simulink model "NLGuidance"  (R2016a)
settings: Solver=ode3  StartTime=0.0  StopTime=10.0  FixedStep=.02  RelTol=1e-3
model workspace (MAT data in the model file):
  F = [0.0104799567177; 0.0105274136759; 0.00258730184958; 0.00112291450915; 0.0065543125439; 0]
  N = 51
  S1 = [2.42464759278 -2.49697623385 -0.253883104432 -3.312058597 3.28063521535 2.42464759278 -2.49697623385 -0.253883104432 -3.312058597 3.28063521535 2.42464759278 -2.49697623385 ... (7515 elements, 5x1503)]
  S2 = [-47.5753524072 -52.4969762338 -50.2538831044 -53.312058597 -46.7193647847 -53.1933464928 -58.0206597562 -53.298625948 -53.0732596071 -45.5277132009 -58.8093605499 -63.5421671216 ... (7515 elements, 5x1503)]
  S3 = [-5.62481372887 -5.52769980874 -3.05143765206 0.237149289911 1.1849461568 -5.61799408553 -5.52368352234 -3.04474284358 0.238798989919 1.19165158379 -5.61601405716 -5.52150736543 ... (7515 elements, 5x1503)]
  S4 = [0 0 0 0 0 0 0 0 0 0 0 0 ... (7515 elements, 5x1503)]
  Vt = [0 0 0 0 0 0 0 0 0 0 0 0 ... (1503 elements, 501x3)]
  Vv = [1.1849461568 1.19165158379 1.19363427504 1.1947051518 1.20742767257 1.21177592763 1.21717805586 1.22205358332 1.22753574851 1.22892415591 1.22911717004 1.25058652202 ... (1503 elements, 501x3)]
  Vvmag = [6.45855507903 6.44973720458 6.44685088198 6.4408859639 6.4366826743 6.42659096353 6.42411891458 6.41278379056 6.40944425236 6.4051659263 6.38964384833 6.38667032718 ... (501 elements, 501x1)]
  X = [2.42464759278  -3.58806283515  -3.13212037163  -4.62859462973  -4.56044848222  -1.58805327826  -4.31562089748  -1.59798361729  3.6518933724  -1.65480947533  1.86919995453  -3.44104646715; -2.49697623385  -3.26410626081  1.1374607513  -4.53307798606  3.16641265871  2.30316995677  -4.22846546614  1.19685177791  4.5962066329  1.482802268  -2.27100282896  -2.50278022892; -0.253883104432  1.58732884776  -3.37955300207  -2.05245406097  -2.56581901551  -2.72520301408  -1.22048178872  -1.58600952642  3.65490458678  1.85411206404  -0.00605968294054  -1.90223108815; -3.312058597  1.68742830515  3.12131217871  1.23610531908  3.08830453111  -2.73426128729  -0.852168562096  1.63529528737  1.04129979322  3.9147593874  -2.83132054006  -1.00180163899; 3.28063521535  1.89810778603  4.32221989343  2.18269243779  -3.3024120093  -2.00531011718  -0.0516837044744  2.44755242786  1.9309412878  5  4.9501252848  -0.842692668272; -3.6978315289  -3.58806283515  1.68549199744  -4.5188954159  -4.66205440883  -1.6875649026  -4.35220746466  1.34311705486  0.811657546537  -1.85555021076  -3.19980711127  -4.38418451801]
  Xap1 = [3.53742766553 3.54841812521 3.55649436401 3.56301032299 3.56900127601 3.57285766144 3.57579889741 3.57816116305 3.57954580685 3.57954139291 3.5792899619 3.58161806007 ... (1503 elements, 501x3)]
  Xap2 = [3.00894026262 2.99947384008 2.99278206158 2.98751350515 2.98264302934 2.97978827516 2.97774180284 2.97617755456 2.97550435147 2.97614326838 2.97696071264 2.97513994677 ... (1503 elements, 501x3)]
  Xr = [10 11.2284720857 12.4539847001 13.6735561742 14.8879723634 16.0937793652 17.2959786101 18.4820399899 19.6645679603 20.8393619799 21.9947001613 23.1446286766 ... (1503 elements, 501x3)]
  Xrmag = [15.65732221 23.8105907731 30.9856356907 38.4540834067 46.0738528973 53.7662892745 61.5065103501 69.2725920166 77.0607192366 84.8582850512 92.6527324163 100.450411961 ... (501 elements, 501x1)]
  Xtarg = [3.28063521535 3.28063521535 3.28063521535 3.28063521535 3.28063521535 3.28063521535 3.28063521535 3.28063521535 3.28063521535 3.28063521535 3.28063521535 3.28063521535 ... (1503 elements, 501x3)]
  Xv = [-46.7193647847 -45.5277132009 -44.3340789258 -43.139373774 -41.9319461015 -40.7201701738 -39.502992118 -38.2809385346 -37.0534027861 -35.8244786302 -34.5953614602 -33.3447749382 ... (1503 elements, 501x3)]
  ans = [0  0  0; 2  2  2; 4  4  4]
  cmd = timeseries
  cmd.DataInfo = tsdata.datametadata
  cmd.DataInfo.Interpolation = tsdata.interpolation
  cmd.DataInfo.Interpolation.Fhandle : function handle (value not decoded)
  cmd.DataInfo.Interpolation.Name = 'zoh'
  cmd.TimeInfo = tsdata.timemetadata
  cmd.TimeInfo.DuplicateTimes = 0
  cmd.TimeInfo.Initialized = 1
  cmd.QualityInfo = tsdata.qualmetadata
  cmd1 = []
  cmd2 = []
  count = 136
  curPath = '/Users/khouloud.gaaloul/Documents/Projects/QRA-Search/Problems/SimulinkTesting'
  curve : matlab.graphics.animation.AnimatedLine (value not decoded)
  curveo = matlab.graphics.animation.AnimatedLine
  curveo.LineWidthMode = 'manual'
  curveo.LineWidth_I = 2
  curveo.CurrentLine_I = 0
  curveo.SegmentContainer_I = matlab.graphics.primitive.world.Group
  curveo.SegmentContainer_I.SerializableChildren = matlab.graphics.internal.AnimatedSegment
  curveo.SegmentContainer_I.SerializableChildren.Edge = matlab.graphics.primitive.world.LineStrip
  curveo.SegmentContainer_I.SerializableChildren.Edge.StripData_I = [1 502]
  curveo.SegmentContainer_I.SerializableChildren.Edge.LineWidth_I = 2
  curveo.SegmentContainer_I.SerializableChildren.Edge.VertexData_I = [3.00894021988 2.64835071564 4.92497825623 2.9994738102 2.63493180275 4.93706846237 2.99278211594 2.62207984924 4.94912099838 2.98751354218 2.61010932922 4.96028995514 ... (1503 elements, 3x501)]
  curveo.SegmentContainer_I.SerializableChildren.Edge.ColorData_I = [0; 0; 0; 255]
  curveo.SegmentContainer_I.SerializableChildren.Edge.ColorBinding_I = 'object'
  curveo.SegmentContainer_I.SerializableChildren.Edge.Description_I = 'AnimatedSegment Edge'
  curveo.SegmentContainer_I.SerializableChildren.Edge.HandleVisibility_I = 'off'
  curveo.SegmentContainer_I.SerializableChildren.Edge.Internal = 1
  curveo.SegmentContainer_I.SerializableChildren.Edge.SerializableApplicationData = struct()
  curveo.SegmentContainer_I.SerializableChildren.Edge.Copyable = 1
  curveo.SegmentContainer_I.SerializableChildren.MarkerHandle = matlab.graphics.primitive.world.Marker
  curveo.SegmentContainer_I.SerializableChildren.MarkerHandle.EdgeColorData_I = [0; 0; 0; 255]
  curveo.SegmentContainer_I.SerializableChildren.MarkerHandle.VertexData_I = [3.00894021988 2.64835071564 4.92497825623 2.9994738102 2.63493180275 4.93706846237 2.99278211594 2.62207984924 4.94912099838 2.98751354218 2.61010932922 4.96028995514 ... (1503 elements, 3x501)]
  curveo.SegmentContainer_I.SerializableChildren.MarkerHandle.PickableParts_I = 'none'
  curveo.SegmentContainer_I.SerializableChildren.MarkerHandle.Description_I = 'AnimatedSegment MarkerHandle'
  curveo.SegmentContainer_I.SerializableChildren.MarkerHandle.Visible_I = 'off'
  curveo.SegmentContainer_I.SerializableChildren.MarkerHandle.HandleVisibility_I = 'off'
  curveo.SegmentContainer_I.SerializableChildren.MarkerHandle.Internal = 1
  curveo.SegmentContainer_I.SerializableChildren.MarkerHandle.SerializableApplicationData = struct()
  curveo.SegmentContainer_I.SerializableChildren.MarkerHandle.Copyable = 1
  curveo.SegmentContainer_I.SerializableChildren.MaxNumPoints_I = 5000
  curveo.SegmentContainer_I.SerializableChildren.XData_I = [3.00894026262 2.99947384008 2.99278206158 2.98751350515 2.98264302934 2.97978827516 2.97774180284 2.97617755456 2.97550435147 2.97614326838 2.97696071264 2.97513994677 ... (5000 elements, 1x5000)]
  curveo.SegmentContainer_I.SerializableChildren.YData_I = [2.64835074056 2.63493178346 2.62207989272 2.61010927833 2.59912240045 2.58878484686 2.57921418375 2.57035768583 2.56215199533 2.55453681534 2.54751560237 2.54111946622 ... (5000 elements, 1x5000)]
  curveo.SegmentContainer_I.SerializableChildren.ZData_I = [4.92497802224 4.93706839336 4.94912096266 4.96029006041 4.97012356487 4.97983400233 4.98881546471 4.99704254051 5.00481819698 5.01242680713 5.01939367699 5.02450802519 ... (5000 elements, 1x5000)]
  curveo.SegmentContainer_I.SerializableChildren.Head_I = 501
  curveo.SegmentContainer_I.SerializableChildren.HitTest_I = 'off'
  curveo.SegmentContainer_I.SerializableChildren.Internal = 0
  curveo.SegmentContainer_I.SerializableChildren.SerializableApplicationData = struct()
  curveo.SegmentContainer_I.SerializableChildren.Copyable = 1
  curveo.SegmentContainer_I.Description_I = 'AnimatedLine SegmentContainer'
  curveo.SegmentContainer_I.HandleVisibility_I = 'off'
  curveo.SegmentContainer_I.Internal = 1
  curveo.SegmentContainer_I.SerializableApplicationData = struct()
  curveo.SegmentContainer_I.Copyable = 1
  curveo.NumPointsAdded_I = 501
  curveo.SerializableBehavior = struct()
  curveo.matlab.graphics.internal.GraphicsCoreProperties.TopLevelSerializedObject = 'on'
  curveo.BeingDeleted = 'off'
  curveo.Annotation = matlab.graphics.eventdata.Annotation
  curveo.Annotation.LegendInformation = matlab.graphics.eventdata.LegendEntry
  curveo.Annotation.Copyable = 1
  curveo.Internal = 0
  curveo.SerializableApplicationData = struct()
  curveo.Copyable = 1
  curvet = matlab.graphics.animation.AnimatedLine
  curvet.LineWidthMode = 'manual'
  curvet.LineWidth_I = 2
  curvet.CurrentLine_I = 0
  curvet.SegmentContainer_I = matlab.graphics.primitive.world.Group
  curvet.SegmentContainer_I.SerializableChildren = matlab.graphics.internal.AnimatedSegment
  curvet.SegmentContainer_I.SerializableChildren.Edge = matlab.graphics.primitive.world.LineStrip
  curvet.SegmentContainer_I.SerializableChildren.Edge.StripData_I = [1 502]
  curvet.SegmentContainer_I.SerializableChildren.Edge.LineWidth_I = 2
  curvet.SegmentContainer_I.SerializableChildren.Edge.VertexData_I = [3.28063511848 1.89810776711 4.32221984863 3.28063511848 1.89810776711 4.32221984863 3.28063511848 1.89810776711 4.32221984863 3.28063511848 1.89810776711 4.32221984863 ... (1503 elements, 3x501)]
  curvet.SegmentContainer_I.SerializableChildren.Edge.ColorData_I = [0; 0; 0; 255]
  curvet.SegmentContainer_I.SerializableChildren.Edge.ColorBinding_I = 'object'
  curvet.SegmentContainer_I.SerializableChildren.Edge.Description_I = 'AnimatedSegment Edge'
  curvet.SegmentContainer_I.SerializableChildren.Edge.HandleVisibility_I = 'off'
  curvet.SegmentContainer_I.SerializableChildren.Edge.Internal = 1
  curvet.SegmentContainer_I.SerializableChildren.Edge.SerializableApplicationData = struct()
  curvet.SegmentContainer_I.SerializableChildren.Edge.Copyable = 1
  curvet.SegmentContainer_I.SerializableChildren.MarkerHandle = matlab.graphics.primitive.world.Marker
  curvet.SegmentContainer_I.SerializableChildren.MarkerHandle.EdgeColorData_I = [0; 0; 0; 255]
  curvet.SegmentContainer_I.SerializableChildren.MarkerHandle.VertexData_I = [3.28063511848 1.89810776711 4.32221984863 3.28063511848 1.89810776711 4.32221984863 3.28063511848 1.89810776711 4.32221984863 3.28063511848 1.89810776711 4.32221984863 ... (1503 elements, 3x501)]
  curvet.SegmentContainer_I.SerializableChildren.MarkerHandle.PickableParts_I = 'none'
  curvet.SegmentContainer_I.SerializableChildren.MarkerHandle.Description_I = 'AnimatedSegment MarkerHandle'
  curvet.SegmentContainer_I.SerializableChildren.MarkerHandle.Visible_I = 'off'
  curvet.SegmentContainer_I.SerializableChildren.MarkerHandle.HandleVisibility_I = 'off'
  curvet.SegmentContainer_I.SerializableChildren.MarkerHandle.Internal = 1
  curvet.SegmentContainer_I.SerializableChildren.MarkerHandle.SerializableApplicationData = struct()
  curvet.SegmentContainer_I.SerializableChildren.MarkerHandle.Copyable = 1
  curvet.SegmentContainer_I.SerializableChildren.MaxNumPoints_I = 5000
  curvet.SegmentContainer_I.SerializableChildren.XData_I = [3.28063521535 3.28063521535 3.28063521535 3.28063521535 3.28063521535 3.28063521535 3.28063521535 3.28063521535 3.28063521535 3.28063521535 3.28063521535 3.28063521535 ... (5000 elements, 1x5000)]
  curvet.SegmentContainer_I.SerializableChildren.YData_I = [1.89810778603 1.89810778603 1.89810778603 1.89810778603 1.89810778603 1.89810778603 1.89810778603 1.89810778603 1.89810778603 1.89810778603 1.89810778603 1.89810778603 ... (5000 elements, 1x5000)]
  curvet.SegmentContainer_I.SerializableChildren.ZData_I = [4.32221989343 4.32221989343 4.32221989343 4.32221989343 4.32221989343 4.32221989343 4.32221989343 4.32221989343 4.32221989343 4.32221989343 4.32221989343 4.32221989343 ... (5000 elements, 1x5000)]
  curvet.SegmentContainer_I.SerializableChildren.Head_I = 501
  curvet.SegmentContainer_I.SerializableChildren.HitTest_I = 'off'
  curvet.SegmentContainer_I.SerializableChildren.Internal = 0
  curvet.SegmentContainer_I.SerializableChildren.SerializableApplicationData = struct()
  curvet.SegmentContainer_I.SerializableChildren.Copyable = 1
  curvet.SegmentContainer_I.Description_I = 'AnimatedLine SegmentContainer'
  curvet.SegmentContainer_I.HandleVisibility_I = 'off'
  curvet.SegmentContainer_I.Internal = 1
  curvet.SegmentContainer_I.SerializableApplicationData = struct()
  curvet.SegmentContainer_I.Copyable = 1
  curvet.NumPointsAdded_I = 501
  curvet.SerializableBehavior = struct()
  curvet.matlab.graphics.internal.GraphicsCoreProperties.TopLevelSerializedObject = 'on'
  curvet.BeingDeleted = 'off'
  curvet.Annotation = matlab.graphics.eventdata.Annotation
  curvet.Annotation.LegendInformation = matlab.graphics.eventdata.LegendEntry
  curvet.Annotation.Copyable = 1
  curvet.Internal = 0
  curvet.SerializableApplicationData = struct()
  curvet.Copyable = 1
  curvev = matlab.graphics.animation.AnimatedLine
  curvev.LineWidthMode = 'manual'
  curvev.LineWidth_I = 2
  curvev.CurrentLine_I = 0
  curvev.SegmentContainer_I = matlab.graphics.primitive.world.Group
  curvev.SegmentContainer_I.SerializableChildren = matlab.graphics.internal.AnimatedSegment
  curvev.SegmentContainer_I.SerializableChildren.Edge = matlab.graphics.primitive.world.LineStrip
  curvev.SegmentContainer_I.SerializableChildren.Edge.StripData_I = [1 502]
  curvev.SegmentContainer_I.SerializableChildren.Edge.LineWidth_I = 2
  curvev.SegmentContainer_I.SerializableChildren.Edge.VertexData_I = [-46.7193641663 -48.101890564 45.6777801514 -45.5277137756 -52.3846321106 48.6807975769 -44.3340797424 -56.6636123657 51.6837692261 -43.1393737793 -60.9370346069 54.6803245544 ... (1503 elements, 3x501)]
  curvev.SegmentContainer_I.SerializableChildren.Edge.ColorData_I = [0; 0; 0; 255]
  curvev.SegmentContainer_I.SerializableChildren.Edge.ColorBinding_I = 'object'
  curvev.SegmentContainer_I.SerializableChildren.Edge.Description_I = 'AnimatedSegment Edge'
  curvev.SegmentContainer_I.SerializableChildren.Edge.HandleVisibility_I = 'off'
  curvev.SegmentContainer_I.SerializableChildren.Edge.Internal = 1
  curvev.SegmentContainer_I.SerializableChildren.Edge.SerializableApplicationData = struct()
  curvev.SegmentContainer_I.SerializableChildren.Edge.Copyable = 1
  curvev.SegmentContainer_I.SerializableChildren.MarkerHandle = matlab.graphics.primitive.world.Marker
  curvev.SegmentContainer_I.SerializableChildren.MarkerHandle.EdgeColorData_I = [0; 0; 0; 255]
  curvev.SegmentContainer_I.SerializableChildren.MarkerHandle.VertexData_I = [-46.7193641663 -48.101890564 45.6777801514 -45.5277137756 -52.3846321106 48.6807975769 -44.3340797424 -56.6636123657 51.6837692261 -43.1393737793 -60.9370346069 54.6803245544 ... (1503 elements, 3x501)]
  curvev.SegmentContainer_I.SerializableChildren.MarkerHandle.PickableParts_I = 'none'
  curvev.SegmentContainer_I.SerializableChildren.MarkerHandle.Description_I = 'AnimatedSegment MarkerHandle'
  curvev.SegmentContainer_I.SerializableChildren.MarkerHandle.Visible_I = 'off'
  curvev.SegmentContainer_I.SerializableChildren.MarkerHandle.HandleVisibility_I = 'off'
  curvev.SegmentContainer_I.SerializableChildren.MarkerHandle.Internal = 1
  curvev.SegmentContainer_I.SerializableChildren.MarkerHandle.SerializableApplicationData = struct()
  curvev.SegmentContainer_I.SerializableChildren.MarkerHandle.Copyable = 1
  curvev.SegmentContainer_I.SerializableChildren.MaxNumPoints_I = 5000
  curvev.SegmentContainer_I.SerializableChildren.XData_I = [-46.7193647847 -45.5277132009 -44.3340789258 -43.139373774 -41.9319461015 -40.7201701738 -39.502992118 -38.2809385346 -37.0534027861 -35.8244786302 -34.5953614602 -33.3447749382 ... (5000 elements, 1x5000)]
  curvev.SegmentContainer_I.SerializableChildren.YData_I = [-48.101892214 -52.3846332875 -56.663611085 -60.93703548 -65.20593249 -69.4668713892 -73.7274049649 -77.9871267457 -82.2407780144 -86.4920761433 -90.7431651505 -94.9853167819 ... (5000 elements, 1x5000)]
  curvev.SegmentContainer_I.SerializableChildren.ZData_I = [45.6777801066 48.680795879 51.6837683233 54.6803231469 57.6757020576 60.666276224 63.6537597154 66.6335569064 69.6091973174 72.5839099026 75.5526555129 78.520090746 ... (5000 elements, 1x5000)]
  curvev.SegmentContainer_I.SerializableChildren.Head_I = 501
  curvev.SegmentContainer_I.SerializableChildren.HitTest_I = 'off'
  curvev.SegmentContainer_I.SerializableChildren.Internal = 0
  curvev.SegmentContainer_I.SerializableChildren.SerializableApplicationData = struct()
  curvev.SegmentContainer_I.SerializableChildren.Copyable = 1
  curvev.SegmentContainer_I.Description_I = 'AnimatedLine SegmentContainer'
  curvev.SegmentContainer_I.HandleVisibility_I = 'off'
  curvev.SegmentContainer_I.Internal = 1
  curvev.SegmentContainer_I.SerializableApplicationData = struct()
  curvev.SegmentContainer_I.Copyable = 1
  curvev.NumPointsAdded_I = 501
  curvev.SerializableBehavior = struct()
  curvev.matlab.graphics.internal.GraphicsCoreProperties.TopLevelSerializedObject = 'on'
  curvev.BeingDeleted = 'off'
  curvev.Annotation = matlab.graphics.eventdata.Annotation
  curvev.Annotation.LegendInformation = matlab.graphics.eventdata.LegendEntry
  curvev.Annotation.Copyable = 1
  curvev.Internal = 0
  curvev.SerializableApplicationData = struct()
  curvev.Copyable = 1
  d = 10
  dev = [0.998411888767 0.99782484185 0.997422855714 0.997059153759 0.99673360256 0.996441028681 0.996174188817 0.995929724086 0.995704685947 0.995496539497 0.995301805204 0.995118534567 ... (501 elements, 501x1)]
  diff = [-0.0110961446926 -0.0111456874882 -0.0111717248678 -0.0112203324043 -0.0112177067868 -0.0112470382447 -0.0112585651595 -0.0112536842015 -0.0112567920009 -0.0112598719834 -0.0112758132864 -0.011238461177 ... (500 elements, 500x1)]
  heado : matlab.graphics.chart.primitive.Scatter (value not decoded)
  headt : matlab.graphics.chart.primitive.Scatter (value not decoded)
  headv : matlab.graphics.chart.primitive.Scatter (value not decoded)
  hws : Simulink.ModelWorkspace (value not decoded)
  i = 26
  inputSize = 6
  j = 3
  list : struct (value not decoded)
  m = [-0.999723895919 -0.999364400237 -0.991672916331 -0.981758345493 -0.98121871348 -0.980992634152 -0.979214833695 -0.97816820181 -0.975813767607 -0.973821424379 -0.973796463479 -0.972935922229 ... (3006 elements, 1002x3)]
  modelpath = '/Users/khouloud.gaaloul/Documents/Projects/QRA-Search/SimulinkModels/4_nlguide/'
  mt = [0.997620134247 0.997296649802 0.994217918569 0.993324313281 0.991703646703 0.985900322398 0.985631450718 0.976402580538 0.973784078633 0.970318825583 0.969896216991 0.965968068121 ... (1503 elements, 501x3)]
  mv = [-0.993370609414 -0.990984924743 -0.989879999798 -0.982454455416 -0.979488128766 -0.978091228792 -0.976254482971 -0.973907633905 -0.96148789861 -0.959724271782 -0.942427931753 -0.941335472094 ... (1503 elements, 501x3)]
  n = 6
  nbrInputs = 4
  nbrTimeSteps = 501
  r2 = 1000000
  s = 4
  simOut = Simulink.SimulationOutput
  simOut.Data.Xap1 = [3.53742766553 3.54841812521 3.55649436401 3.56301032299 3.56900127601 3.57285766144 3.57579889741 3.57816116305 3.57954580685 3.57954139291 3.5792899619 3.58161806007 ... (1503 elements, 501x3)]
  simOut.Data.Xap2 = [3.00894026262 2.99947384008 2.99278206158 2.98751350515 2.98264302934 2.97978827516 2.97774180284 2.97617755456 2.97550435147 2.97614326838 2.97696071264 2.97513994677 ... (1503 elements, 501x3)]
  simOut.Data.Xr = timeseries
  simOut.Data.Xr.DataInfo = tsdata.datametadata
  simOut.Data.Xr.DataInfo.Interpolation = tsdata.interpolation
  simOut.Data.Xr.DataInfo.Interpolation.Fhandle : function handle (value not decoded)
  simOut.Data.Xr.DataInfo.Interpolation.Name = 'zoh'
  simOut.Data.Xr.TimeInfo = tsdata.timemetadata
  simOut.Data.Xr.TimeInfo.DuplicateTimes = 0
  simOut.Data.Xr.TimeInfo.Initialized = 1
  simOut.Data.Xr.QualityInfo = tsdata.qualmetadata
  simOut.Data.cmd1 = []
  simOut.Data.cmd2 = []
  simOut.Data.k = timeseries
  simOut.Data.k.Name = 'k'
  simOut.Data.k.DataInfo = tsdata.datametadata
  simOut.Data.k.DataInfo.Interpolation = tsdata.interpolation
  simOut.Data.k.DataInfo.Interpolation.Fhandle : function handle (value not decoded)
  simOut.Data.k.DataInfo.Interpolation.Name = 'zoh'
  simOut.Data.k.TimeInfo = tsdata.timemetadata
  simOut.Data.k.TimeInfo.DuplicateTimes = 0
  simOut.Data.k.TimeInfo.Initialized = 1
  simOut.Data.k.QualityInfo = tsdata.qualmetadata
  simOut.Data.tout = [0 0.02 0.04 0.06 0.08 0.1 0.12 0.14 0.16 0.18 0.2 0.22 ... (501 elements, 501x1)]
  simOut.Data.varout.time = [0 0.02 0.04 0.06 0.08 0.1 0.12 0.14 0.16 0.18 0.2 0.22 ... (501 elements, 501x1)]
  simOut.Data.varout.signals.values = [3.00894026262 2.99947384008 2.99278206158 2.98751350515 2.98264302934 2.97978827516 2.97774180284 2.97617755456 2.97550435147 2.97614326838 2.97696071264 2.97513994677 ... (1503 elements, 501x3)]
  simOut.Data.varout.signals.dimensions = 3
  simOut.Data.varout.signals.label = ''
  simOut.Data.varout.signals.blockName = 'NLGuidance/yout'
  simOut.Metadata = Simulink.SimulationMetadata
  simOut.Metadata.ModelInfo.ModelName = 'NLGuidance'
  simOut.Metadata.ModelInfo.ModelVersion = '1.71'
  simOut.Metadata.ModelInfo.ModelFilePath = '/Users/khouloud.gaaloul/Documents/Projects/QRA-Search/SimulinkModels/4_nlguide/NLGuidance.slx'
  simOut.Metadata.ModelInfo.UserID = 'khouloud.gaaloul'
  simOut.Metadata.ModelInfo.MachineName = ''
  simOut.Metadata.ModelInfo.Platform = 'MACI64'
  simOut.Metadata.ModelInfo.ModelStructuralChecksum = [499275200; 701238149; 2662302127; 2261484637]
  simOut.Metadata.ModelInfo.SimulationMode = 'normal'
  simOut.Metadata.ModelInfo.StartTime = 0
  simOut.Metadata.ModelInfo.StopTime = 10
  simOut.Metadata.ModelInfo.SolverInfo.Type = 'Fixed-Step'
  simOut.Metadata.ModelInfo.SolverInfo.Solver = 'FixedStepDiscrete'
  simOut.Metadata.ModelInfo.SolverInfo.FixedStepSize = 0.02
  simOut.Metadata.ModelInfo.SimulinkVersion.Name = 'Simulink'
  simOut.Metadata.ModelInfo.SimulinkVersion.Version = '8.7'
  simOut.Metadata.ModelInfo.SimulinkVersion.Release = '(R2016a)'
  simOut.Metadata.ModelInfo.SimulinkVersion.Date = '10-Feb-2016'
  simOut.Metadata.TimingInfo.WallClockTimestampStart = '2018-03-23 12:06:35.158343'
  simOut.Metadata.TimingInfo.WallClockTimestampStop = '2018-03-23 12:06:35.767810'
  simOut.Metadata.TimingInfo.InitializationElapsedWallTime = 0.558519
  simOut.Metadata.TimingInfo.ExecutionElapsedWallTime = 0.005275
  simOut.Metadata.TimingInfo.TerminationElapsedWallTime = 0.04569
  simOut.Metadata.TimingInfo.TotalElapsedWallTime = 0.609484
  simOut.Metadata.ExecutionInfo.StopEvent = 'ReachedStopTime'
  simOut.Metadata.ExecutionInfo.StopEventSource = []
  simOut.Metadata.ExecutionInfo.StopEventDescription = 'Reached stop time of 10'
  simOut.Metadata.ExecutionInfo.ErrorDiagnostic = []
  simOut.Metadata.ExecutionInfo.WarningDiagnostics(1).Diagnostic = MSLDiagnostic
  simOut.Metadata.ExecutionInfo.WarningDiagnostics(1).Diagnostic.identifier = 'Simulink:blocks:MatchingFromNotFound'
  simOut.Metadata.ExecutionInfo.WarningDiagnostics(1).Diagnostic.message = 'Matching "From" for "Goto" ''<a href="matlab:open_and_hilite_hyperlink (''NLGuidance/NLGuidance/Goto4'',''error'')">NLGuidance/NLGuidance/Goto4</a>'' not found'
  simOut.Metadata.ExecutionInfo.WarningDiagnostics(1).Diagnostic.paths = {'NLGuidance/NLGuidance/Goto4'}
  simOut.Metadata.ExecutionInfo.WarningDiagnostics(1).Diagnostic.arguments = {'NLGuidance/NLGuidance/Goto4'}
  simOut.Metadata.ExecutionInfo.WarningDiagnostics(1).SimulationPhase = 'Initialization'
  simOut.Metadata.ExecutionInfo.WarningDiagnostics(1).SimulationTime = []
  simOut.Metadata.ExecutionInfo.WarningDiagnostics(2).Diagnostic = MSLDiagnostic
  simOut.Metadata.ExecutionInfo.WarningDiagnostics(2).Diagnostic.identifier = 'Simulink:blocks:MatchingFromNotFound'
  simOut.Metadata.ExecutionInfo.WarningDiagnostics(2).Diagnostic.message = 'Matching "From" for "Goto" ''<a href="matlab:open_and_hilite_hyperlink (''NLGuidance/NLGuidance/Outer/Goto'',''error'')">NLGuidance/NLGuidance/Outer/Goto</a>'' not found'
  simOut.Metadata.ExecutionInfo.WarningDiagnostics(2).Diagnostic.paths = {'NLGuidance/NLGuidance/Outer/Goto'}
  simOut.Metadata.ExecutionInfo.WarningDiagnostics(2).Diagnostic.arguments = {'NLGuidance/NLGuidance/Outer/Goto'}
  simOut.Metadata.ExecutionInfo.WarningDiagnostics(2).SimulationPhase = 'Initialization'
  simOut.Metadata.ExecutionInfo.WarningDiagnostics(2).SimulationTime = []
  simOut.Metadata.ExecutionInfo.WarningDiagnostics(3).Diagnostic = MSLDiagnostic
  simOut.Metadata.ExecutionInfo.WarningDiagnostics(3).Diagnostic.identifier = 'Simulink:blocks:MatchingFromNotFound'
  simOut.Metadata.ExecutionInfo.WarningDiagnostics(3).Diagnostic.message = 'Matching "From" for "Goto" ''<a href="matlab:open_and_hilite_hyperlink (''NLGuidance/NLGuidance/Outer/Goto11'',''error'')">NLGuidance/NLGuidance/Outer/Goto11</a>'' not found'
  simOut.Metadata.ExecutionInfo.WarningDiagnostics(3).Diagnostic.paths = {'NLGuidance/NLGuidance/Outer/Goto11'}
  simOut.Metadata.ExecutionInfo.WarningDiagnostics(3).Diagnostic.arguments = {'NLGuidance/NLGuidance/Outer/Goto11'}
  simOut.Metadata.ExecutionInfo.WarningDiagnostics(3).SimulationPhase = 'Initialization'
  simOut.Metadata.ExecutionInfo.WarningDiagnostics(3).SimulationTime = []
  simOut.Metadata.ExecutionInfo.WarningDiagnostics(4).Diagnostic = MSLDiagnostic
  simOut.Metadata.ExecutionInfo.WarningDiagnostics(4).Diagnostic.identifier = 'Simulink:blocks:MatchingFromNotFound'
  simOut.Metadata.ExecutionInfo.WarningDiagnostics(4).Diagnostic.message = 'Matching "From" for "Goto" ''<a href="matlab:open_and_hilite_hyperlink (''NLGuidance/NLGuidance/Outer/Goto12'',''error'')">NLGuidance/NLGuidance/Outer/Goto12</a>'' not found'
  simOut.Metadata.ExecutionInfo.WarningDiagnostics(4).Diagnostic.paths = {'NLGuidance/NLGuidance/Outer/Goto12'}
  simOut.Metadata.ExecutionInfo.WarningDiagnostics(4).Diagnostic.arguments = {'NLGuidance/NLGuidance/Outer/Goto12'}
  simOut.Metadata.ExecutionInfo.WarningDiagnostics(4).SimulationPhase = 'Initialization'
  simOut.Metadata.ExecutionInfo.WarningDiagnostics(4).SimulationTime = []
  simOut.Metadata.ExecutionInfo.WarningDiagnostics(5).Diagnostic = MSLDiagnostic
  simOut.Metadata.ExecutionInfo.WarningDiagnostics(5).Diagnostic.identifier = 'Simulink:blocks:MatchingFromNotFound'
  simOut.Metadata.ExecutionInfo.WarningDiagnostics(5).Diagnostic.message = 'Matching "From" for "Goto" ''<a href="matlab:open_and_hilite_hyperlink (''NLGuidance/NLGuidance/Outer/Goto15'',''error'')">NLGuidance/NLGuidance/Outer/Goto15</a>'' not found'
  simOut.Metadata.ExecutionInfo.WarningDiagnostics(5).Diagnostic.paths = {'NLGuidance/NLGuidance/Outer/Goto15'}
  simOut.Metadata.ExecutionInfo.WarningDiagnostics(5).Diagnostic.arguments = {'NLGuidance/NLGuidance/Outer/Goto15'}
  simOut.Metadata.ExecutionInfo.WarningDiagnostics(5).SimulationPhase = 'Initialization'
  simOut.Metadata.ExecutionInfo.WarningDiagnostics(5).SimulationTime = []
  simOut.Metadata.ExecutionInfo.WarningDiagnostics(6).Diagnostic = MSLDiagnostic
  simOut.Metadata.ExecutionInfo.WarningDiagnostics(6).Diagnostic.identifier = 'Simulink:blocks:MatchingFromNotFound'
  simOut.Metadata.ExecutionInfo.WarningDiagnostics(6).Diagnostic.message = 'Matching "From" for "Goto" ''<a href="matlab:open_and_hilite_hyperlink (''NLGuidance/NLGuidance/Outer/Goto2'',''error'')">NLGuidance/NLGuidance/Outer/Goto2</a>'' not found'
  simOut.Metadata.ExecutionInfo.WarningDiagnostics(6).Diagnostic.paths = {'NLGuidance/NLGuidance/Outer/Goto2'}
  simOut.Metadata.ExecutionInfo.WarningDiagnostics(6).Diagnostic.arguments = {'NLGuidance/NLGuidance/Outer/Goto2'}
  simOut.Metadata.ExecutionInfo.WarningDiagnostics(6).SimulationPhase = 'Initialization'
  simOut.Metadata.ExecutionInfo.WarningDiagnostics(6).SimulationTime = []
  simOut.Metadata.AppInfo = struct()
  sumOut = 1.13428583934e-06
  sumVl = 16.4352757808
  t = 501
  var.time = [0 0.02 0.04 0.06 0.08 0.1 0.12 0.14 0.16 0.18 0.2 0.22 ... (501 elements, 1x501)]
  var.signals(1).values = [-3.6978315289 -3.6978315289 -3.6978315289 -3.6978315289 -3.6978315289 -3.6978315289 -3.6978315289 -3.6978315289 -3.6978315289 -3.6978315289 -3.6978315289 -3.6978315289 ... (1503 elements, 501x3)]
  var.signals(1).dimensions = 3
  var.signals(2).values = [-53.6978315289 -59.2077118695 -64.7164872852 -70.2178371566 -75.7162207012 -81.2132073459 -86.7083572448 -92.2011602946 -97.6815436091 -103.160163297 -108.621486644 -114.081717532 ... (1503 elements, 501x3)]
  var.signals(2).dimensions = 3
  var.signals(3).values = [-5.51226602532 -5.50988034065 -5.5087754157 -5.50134987132 -5.49838354467 -5.4969866447 -5.49514989888 -5.49280304981 -5.48038331451 -5.47861968769 -5.46132334766 -5.460230888 ... (1503 elements, 501x3)]
  var.signals(3).dimensions = 3
  var.signals(4).values = [0 0 0 0 0 0 0 0 0 0 0 0 ... (1503 elements, 501x3)]
  var.signals(4).dimensions = 3
  var.signals(5).values = [1; 1; 1; 1; 1; 1; 1; 1; 1; 1; 1; 1; 1; 1; 1; 1; 1; 1; 1; 1; 1; 1; 1; 1; 1; 1; 1; 1; 1; 1; 1; 1; 1; 1; 1; 1; 1; 1; 1; 1; 1; 1; 1; 1; 1; 1; 1; 1; 1; 1; 1; 1; 1; 1; 1; 1; 1; 1; 1; 1; 1; 1; 1; 1; 1; 1; 1; 1; 1; 1; 1; 1; 1; 1; 1; 1; 1; 1; 1; 1; 1; 1; 1; 1; 1; 1; 1; 1; 1; 1; 1; 1; 1; 1; 1; 1; 1; 1; 1; 1; 1; 1; 1; 1; 1; 1; 1; 1; 1; 1; 1; 1; 1; 1; 1; 1; 1; 1; 1; 1; 1; 1; 1; 1; 1; 1; 1; 1; 1; 1; 1; 1; 1; 1; 1; 1; 1; 1; 1; 1; 1; 1; 1; 1; 1; 1; 1; 1; 1; 1; 1; 1; 1; 1; 1; 1; 1; 1; 1; 1; 1; 1; 1; 1; 1; 1; 1; 1; 1; 1; 1; 1; 1; 1; 1; 1; 1; 1; 1; 1; 1; 1; 1; 1; 1; 1; 1; 1; 1; 1; 1; 1; 1; 1; 1; 1; 1; 1; 1; 1; 1; 1; 1; 1; 1; 1; 1; 1; 1; 1; 1; 1; 1; 1; 1; 1; 1; 1; 1; 1; 1; 1; 1; 1; 1; 1; 1; 1; 1; 1; 1; 1; 1; 1; 1; 1; 1; 1; 1; 1; 1; 1; 1; 1; 1; 1; 1; 1; 1; 1; 1; 1; 1; 1; 1; 1; 1; 1; 1; 1; 1; 1; 1; 1; 1; 1; 1; 1; 1; 1; 1; 1; 1; 1; 1; 1; 1; 1; 1; 1; 1; 1; 1; 1; 1; 1; 1; 1; 1; 1; 1; 1; 1; 1; 1; 1; 1; 1; 1; 1; 1; 1; 1; 1; 1; 1; 1; 1; 1; 1; 1; 1; 1; 1; 1; 1; 1; 1; 1; 1; 1; 1; 1; 1; 1; 1; 1; 1; 1; 1; 1; 1; 1; 1; 1; 1; 1; 1; 1; 1; 1; 1; 1; 1; 1; 1; 1; 1; 1; 1; 1; 1; 1; 1; 1; 1; 1; 1; 1; 1; 1; 1; 1; 1; 1; 1; 1; 1; 1; 1; 1; 1; 1; 1; 1; 1; 1; 1; 1; 1; 1; 1; 1; 1; 1; 1; 1; 1; 1; 1; 1; 1; 1; 1; 1; 1; 1; 1; 1; 1; 1; 1; 1; 1; 1; 1; 1; 1; 1; 1; 1; 1; 1; 1; 1; 1; 1; 1; 1; 1; 1; 1; 1; 1; 1; 1; 1; 1; 1; 1; 1; 1; 1; 1; 1; 1; 1; 1; 1; 1; 1; 1; 1; 1; 1; 1; 1; 1; 1; 1; 1; 1; 1; 1; 1; 1; 1; 1; 1; 1; 1; 1; 1; 1; 1; 1; 1; 1; 1; 1; 1; 1; 1; 1; 1; 1; 1; 1; 1; 1; 1; 1; 1; 1; 1; 1; 1; 1; 1; 1; 1; 1; 1; 1; 1; 1; 1; 1; 1; 1; 1]
  var.signals(5).dimensions = 1
  varout.time = [0 0.02 0.04 0.06 0.08 0.1 0.12 0.14 0.16 0.18 0.2 0.22 ... (501 elements, 501x1)]
  varout.signals.values = [3.00894026262 2.99947384008 2.99278206158 2.98751350515 2.98264302934 2.97978827516 2.97774180284 2.97617755456 2.97550435147 2.97614326838 2.97696071264 2.97513994677 ... (1503 elements, 501x3)]
  varout.signals.dimensions = 3
  varout.signals.label = ''
  varout.signals.blockName = 'NLGuidance/yout'
  x = [2.7049904163 8.31847210292 14.0416550116 19.9218605512 25.7958831948 31.6629046774 37.5137196427 43.3342242648 49.1594101201 54.9752404562 60.7952146721 66.6155429658 ... (501 elements, 501x1)]
  xo = [3.00894026262 2.99947384008 2.99278206158 2.98751350515 2.98264302934 2.97978827516 2.97774180284 2.97617755456 2.97550435147 2.97614326838 2.97696071264 2.97513994677 ... (501 elements, 501x1)]
  xt = [3.28063521535 3.28063521535 3.28063521535 3.28063521535 3.28063521535 3.28063521535 3.28063521535 3.28063521535 3.28063521535 3.28063521535 3.28063521535 3.28063521535 ... (501 elements, 501x1)]
  xv = [-46.7193647847 -45.5277132009 -44.3340789258 -43.139373774 -41.9319461015 -40.7201701738 -39.502992118 -38.2809385346 -37.0534027861 -35.8244786302 -34.5953614602 -33.3447749382 ... (501 elements, 501x1)]
  y = [3.6883959876 9.17834089576 14.9294898906 19.9030920073 24.7285315288 29.5033134454 34.2547577046 38.9972499457 43.7096979702 48.4166380479 53.1197368616 57.8142423866 ... (501 elements, 501x1)]
  yo = [2.64835074056 2.63493178346 2.62207989272 2.61010927833 2.59912240045 2.58878484686 2.57921418375 2.57035768583 2.56215199533 2.55453681534 2.54751560237 2.54111946622 ... (501 elements, 501x1)]
  yout = [3.00894026262 2.99947384008 2.99278206158 2.98751350515 2.98264302934 2.97978827516 2.97774180284 2.97617755456 2.97550435147 2.97614326838 2.97696071264 2.97513994677 ... (1503 elements, 501x3)]
  yt = [1.89810778603 1.89810778603 1.89810778603 1.89810778603 1.89810778603 1.89810778603 1.89810778603 1.89810778603 1.89810778603 1.89810778603 1.89810778603 1.89810778603 ... (501 elements, 501x1)]
  yv = [-48.101892214 -52.3846332875 -56.663611085 -60.93703548 -65.20593249 -69.4668713892 -73.7274049649 -77.9871267457 -82.2407780144 -86.4920761433 -90.7431651505 -94.9853167819 ... (501 elements, 501x1)]
  z = [4.49604856588 6.72999883369 12.0965927953 17.1688972661 22.1258781778 27.0326381497 31.9068218628 36.7791547029 41.639146818 46.4962544595 51.3440742559 56.1827474075 ... (501 elements, 501x1)]
  zo = [4.92497802224 4.93706839336 4.94912096266 4.96029006041 4.97012356487 4.97983400233 4.98881546471 4.99704254051 5.00481819698 5.01242680713 5.01939367699 5.02450802519 ... (501 elements, 501x1)]
  zt = [4.32221989343 4.32221989343 4.32221989343 4.32221989343 4.32221989343 4.32221989343 4.32221989343 4.32221989343 4.32221989343 4.32221989343 4.32221989343 4.32221989343 ... (501 elements, 501x1)]
  zv = [45.6777801066 48.680795879 51.6837683233 54.6803231469 57.6757020576 60.666276224 63.6537597154 66.6335569064 69.6091973174 72.5839099026 75.5526555129 78.520090746 ... (501 elements, 501x1)]
(part 1 of 2)
settings Model: Creator=elliocm  LastModifiedBy=khouloud.gaaloul
settings DataIOCC: ExternalInput=var  LimitDataPoints=on  LoadExternalInput=on  SaveFormat=StructureWithTime  SignalLoggingSaveFormat=ModelDataLogs
settings OptimizationCC: ExpressionDepthLimit=2147483647
settings DebuggingCC: UnderspecifiedInitializationDetection=Classic  MergeDetectMultiDrivingBlocksExec=none  SolverPrmCheckMsg=warning  MultiTaskDSMMsg=warning  MultiTaskCondExecSysMsg=none  StateNameClashWarn=warning
settings HardwareCC: ProdBitPerPointer=32  ProdLargestAtomicFloat=None  ProdIntDivRoundTo=Undefined  ProdEndianess=Unspecified  ProdWordSize=32  ProdHWDeviceType=32-bit Generic
settings ModelReferenceCC: PropagateSignalLabelsOutOfModel=off
settings ConfigComp: CovModelRefEnable=Off

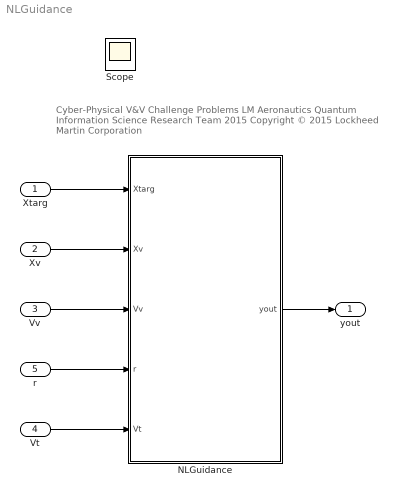
== system NLGuidance ==
  note: Cyber-Physical V&V Challenge Problems
      | LM Aeronautics Quantum Information Science Research Team 2015
      | Copyright © 2015 Lockheed Martin Corporation
  Xtarg : Inport  OutDataTypeStr=double  PortDimensions=3
  Xv : Inport  Port=2  OutDataTypeStr=double  PortDimensions=3
  Vv : Inport  Port=3  OutDataTypeStr=double  PortDimensions=3
  Vt : Inport  Port=4  OutDataTypeStr=double  PortDimensions=3
  r : Inport  Port=5  OutDataTypeStr=double
  NLGuidance : Subsystem
  yout : Outport
  Scope : Scope
  wires:
  NLGuidance/1(yout) -> yout/1
  Xtarg/1 -> NLGuidance/1(Xtarg)
  Xv/1 -> NLGuidance/2(Xv)
  Vv/1 -> NLGuidance/3(Vv)
  r/1 -> NLGuidance/4(r)
  Vt/1 -> NLGuidance/5(Vt)
